simulink model "PID_S_shape_tunning"  (R2023a)
settings: Solver=VariableStepAuto  StartTime=0.0  StopTime=50  RelTol=1e-3
settings Model: Creator=mazen  LastModifiedBy=mazen

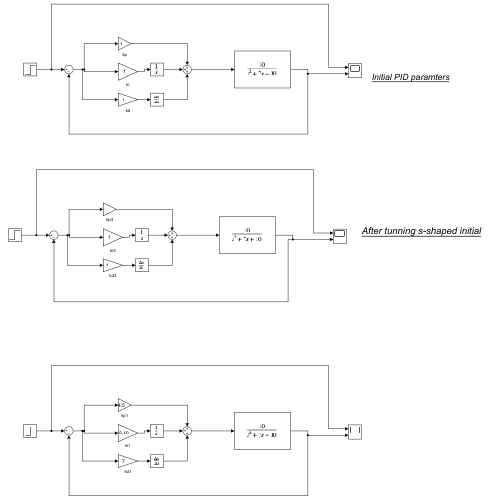
[thumbnail: Simulink's stored preview of the top-level diagram]
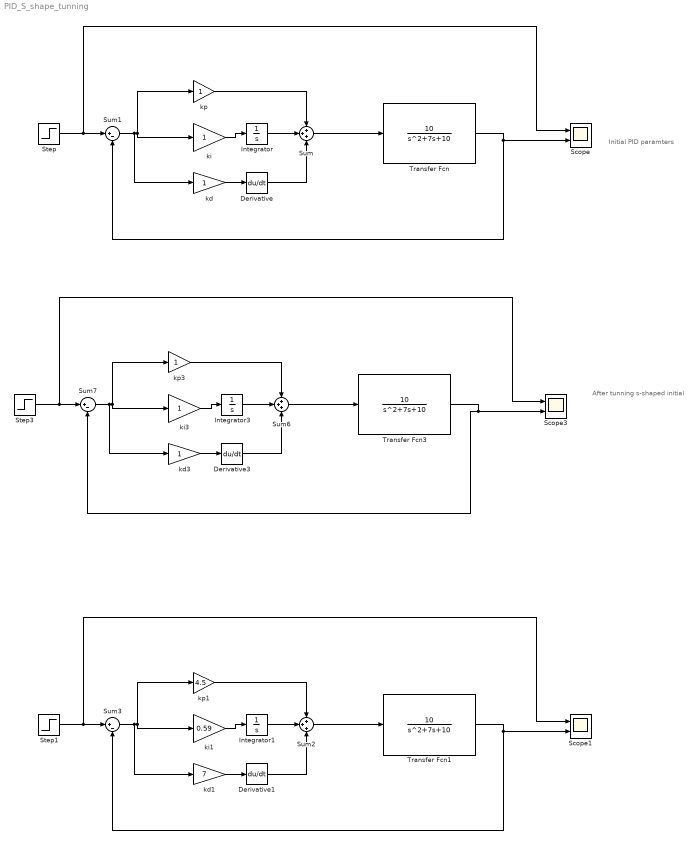
== system PID_S_shape_tunning ==
  note: After tunning s-shaped initial
  note: Initial PID paramters
  Derivative : Derivative
  Derivative1 : Derivative
  Derivative3 : Derivative
  Integrator : Integrator
  Integrator1 : Integrator
  Integrator3 : Integrator
  Scope : Scope  NumInputPorts=2
  Scope1 : Scope  NumInputPorts=2
  Scope3 : Scope  NumInputPorts=2
  Step : Step  SampleTime=0
  Step1 : Step  SampleTime=0
  Step3 : Step  SampleTime=0
  Sum : Sum  Inputs=+++
  Sum1 : Sum  Inputs=|+-
  Sum2 : Sum  Inputs=+++
  Sum3 : Sum  Inputs=|+-
  Sum6 : Sum  Inputs=+++
  Sum7 : Sum  Inputs=|+-
  Transfer Fcn : TransferFcn  Numerator=[10]  Denominator=[1 7 10]
  Transfer Fcn1 : TransferFcn  Numerator=[10]  Denominator=[1 7 10]
  Transfer Fcn3 : TransferFcn  Numerator=[10]  Denominator=[1 7 10]
  kd : Gain
  kd1 : Gain  Gain=7
  kd3 : Gain
  ki : Gain
  ki1 : Gain  Gain=0.59
  ki3 : Gain
  kp : Gain
  kp1 : Gain  Gain=4.5
  kp3 : Gain
  wires:
  kd/1 -> Derivative/1
  ki/1 -> Integrator/1
  Integrator/1 -> Sum/2
  Derivative/1 -> Sum/3
  kp/1 -> Sum/1
  Sum/1 -> Transfer Fcn/1
  Sum1/1 -> kd/1, kp/1, ki/1
  Transfer Fcn/1 -> Scope/2, Sum1/2
  Step/1 -> Scope/1, Sum1/1
  Step1/1 -> Sum3/1, Scope1/1
  Transfer Fcn1/1 -> Sum3/2, Scope1/2
  Sum3/1 -> ki1/1, kp1/1, kd1/1
  Sum2/1 -> Transfer Fcn1/1
  kp1/1 -> Sum2/1
  Derivative1/1 -> Sum2/3
  Integrator1/1 -> Sum2/2
  ki1/1 -> Integrator1/1
  kd1/1 -> Derivative1/1
  kd3/1 -> Derivative3/1
  ki3/1 -> Integrator3/1
  Integrator3/1 -> Sum6/2
  Derivative3/1 -> Sum6/3
  kp3/1 -> Sum6/1
  Sum6/1 -> Transfer Fcn3/1
  Sum7/1 -> kd3/1, kp3/1, ki3/1
  Transfer Fcn3/1 -> Scope3/2, Sum7/2
  Step3/1 -> Scope3/1, Sum7/1
